simulink model "URM_IGM_2b"  (R2014a)
settings: Solver=ode45  StartTime=0.0  StopTime=inf  RelTol=1e-3
values from neighbouring files (symbols this model uses):
  a1 = 2    [URM_SP.m]
  a2 = 1.5    [URM_SP.m]
  a3 = 0.5    [URM_SP.m]
  D = linspace(d1,d2,n)    [URM_SP.m]
libraries: mblibv1 x12, simulink x3
settings Model: Creator=kajak_000  LastModifiedBy=kajak_000
settings SimMechanicsCC: VisDuringSimulation=on

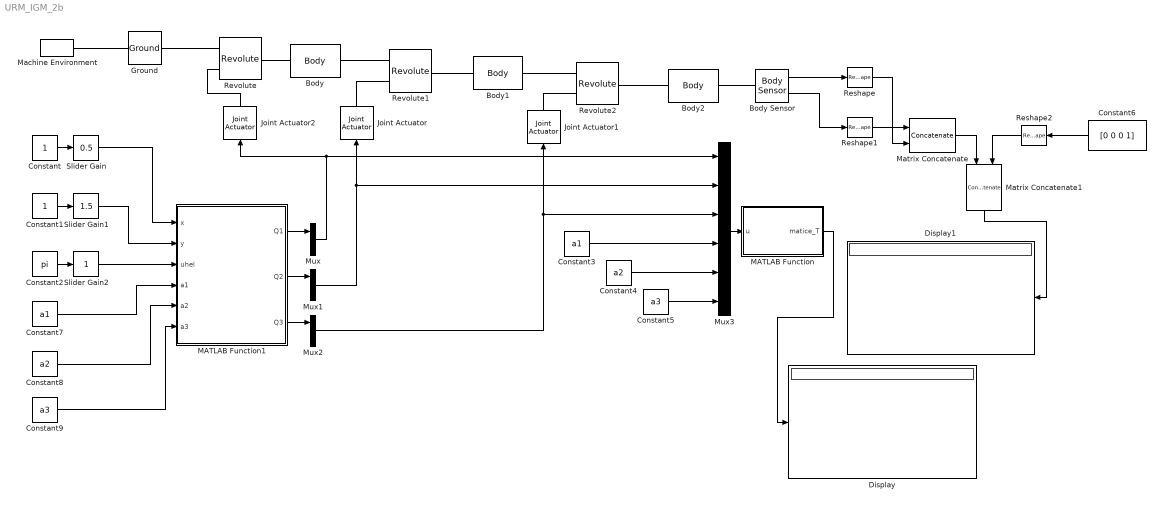
== system URM_IGM_2b ==
  Body : mblibv1/Bodies/Body  LConnTagsString=CS1  RConnTagsString=CS2  UpdateFromCAD=off  DialogClass=MechanicalBodyBlock  Mass=1  MassUnits=kg  InertiaUnits=kg*m^2  Inertia=eye(3)  Shape=Cylinder  ShapeDims=[1 1]  ShapeUnits=m  ShapeUse=false  Density=1  DensityUnits=kg/m^3  DensityUse=false  GraphicsMode=MACHINE_DEFAULT  BodyColorSelMode=MACHINE_DEFAULT  BodyColor=[1 0 0]  AttachedToCS=CG  CG=Left$CG$rameno1.CG$WORLD$WORLD$m$[0 0 0]$Euler X-Y-Z$deg$WORLD$false$none  WorkingFrames=Left$CS1$rameno1.A$World$World$m$[0 0 0]$Euler X-Y-Z$deg$WORLD$true$none#Right$CS2$rameno1.B$World$World$m$[0 0 0]$Euler X-Y-Z$deg$WORLD$true$none  CGPos=rameno1.CG  CGRot=[0 0 0]  CS0Pos=[]  CS0Rot=[]  CS1Pos=rameno1.A  CS1Rot=[0 0 0]  CS2Pos=rameno1.B  CS2Rot=[0 0 0]  CS3Pos=[]  CS3Rot=[]  CS4Pos=[]  CS4Rot=[]  CS5Pos=[]  CS5Rot=[]  CS6Pos=[]  CS6Rot=[]  CS7Pos=[]  CS7Rot=[]  CS8Pos=[]  CS8Rot=[]  CS9Pos=[]  CS9Rot=[]  CS10Pos=[]  CS10Rot=[]  CS11Pos=[]  CS11Rot=[]  CS12Pos=[]  CS12Rot=[]  CS13Pos=[]  CS13Rot=[]  CS14Pos=[]  CS14Rot=[]  CS15Pos=[]  CS15Rot=[]  CS16Pos=[]  CS16Rot=[]  CS17Pos=[]  CS17Rot=[]  CS18Pos=[]  CS18Rot=[]  CS19Pos=[]  CS19Rot=[]  CS20Pos=[]  CS20Rot=[]
  Body Sensor : mblibv1/Sensors &  Actuators/Body Sensor  UpdateFromCAD=off  PhysicalDomain=Mechanical  PortType=blob  Muxed=off  Pose=on  Angle=on  AngleUnits=deg  ArcVelocity=off  ArcVelocityUnits=deg/s  ArcAcceleration=off  ArcAccelerationUnits=deg/s^2  CoordPosition=on  CoordPositionUnits=m  Velocity=off  VelocityUnits=m/s  Acceleration=off  AccelerationUnits=m/s^2  Quaternion=on  QuaternionDT=off  QuaternionDDT=off  QuaternionUnits=off  OutputVector=[1]  ActiveIO=on  Width=12  DialogClass=MechanicalSensorBlock  ReferenceFrame=Absolute (World)
  Body1 : mblibv1/Bodies/Body  LConnTagsString=CS1  RConnTagsString=CS2  UpdateFromCAD=off  DialogClass=MechanicalBodyBlock  Mass=1  MassUnits=kg  InertiaUnits=kg*m^2  Inertia=eye(3)  Shape=Cylinder  ShapeDims=[1 1]  ShapeUnits=m  ShapeUse=false  Density=1  DensityUnits=kg/m^3  DensityUse=false  GraphicsMode=MACHINE_DEFAULT  BodyColorSelMode=MACHINE_DEFAULT  BodyColor=[1 0 0]  AttachedToCS=CG  CG=Left$CG$rameno2.CG$WORLD$WORLD$m$[0 0 0]$Euler X-Y-Z$deg$WORLD$false$none  WorkingFrames=Left$CS1$rameno2.A$World$World$m$[0 0 0]$Euler X-Y-Z$deg$WORLD$true$none#Right$CS2$rameno2.B$World$World$m$[0 0 0]$Euler X-Y-Z$deg$WORLD$true$none  CGPos=rameno2.CG  CGRot=[0 0 0]  CS0Pos=[]  CS0Rot=[]  CS1Pos=rameno2.A  CS1Rot=[0 0 0]  CS2Pos=rameno2.B  CS2Rot=[0 0 0]  CS3Pos=[]  CS3Rot=[]  CS4Pos=[]  CS4Rot=[]  CS5Pos=[]  CS5Rot=[]  CS6Pos=[]  CS6Rot=[]  CS7Pos=[]  CS7Rot=[]  CS8Pos=[]  CS8Rot=[]  CS9Pos=[]  CS9Rot=[]  CS10Pos=[]  CS10Rot=[]  CS11Pos=[]  CS11Rot=[]  CS12Pos=[]  CS12Rot=[]  CS13Pos=[]  CS13Rot=[]  CS14Pos=[]  CS14Rot=[]  CS15Pos=[]  CS15Rot=[]  CS16Pos=[]  CS16Rot=[]  CS17Pos=[]  CS17Rot=[]  CS18Pos=[]  CS18Rot=[]  CS19Pos=[]  CS19Rot=[]  CS20Pos=[]  CS20Rot=[]
  Body2 : mblibv1/Bodies/Body  LConnTagsString=CS1  RConnTagsString=CS2  UpdateFromCAD=off  DialogClass=MechanicalBodyBlock  Mass=1  MassUnits=kg  InertiaUnits=kg*m^2  Inertia=eye(3)  Shape=Cylinder  ShapeDims=[1 1]  ShapeUnits=m  ShapeUse=false  Density=1  DensityUnits=kg/m^3  DensityUse=false  GraphicsMode=MACHINE_DEFAULT  BodyColorSelMode=MACHINE_DEFAULT  BodyColor=[1 0 0]  AttachedToCS=CG  CG=Left$CG$rameno3.CG$WORLD$WORLD$m$[0 0 0]$Euler X-Y-Z$deg$WORLD$false$none  WorkingFrames=Left$CS1$rameno3.A$World$World$m$[0 0 0]$Euler X-Y-Z$deg$WORLD$true$none#Right$CS2$rameno3.B$World$World$m$[0 0 0]$Euler X-Y-Z$deg$WORLD$true$none  CGPos=rameno3.CG  CGRot=[0 0 0]  CS0Pos=[]  CS0Rot=[]  CS1Pos=rameno3.A  CS1Rot=[0 0 0]  CS2Pos=rameno3.B  CS2Rot=[0 0 0]  CS3Pos=[]  CS3Rot=[]  CS4Pos=[]  CS4Rot=[]  CS5Pos=[]  CS5Rot=[]  CS6Pos=[]  CS6Rot=[]  CS7Pos=[]  CS7Rot=[]  CS8Pos=[]  CS8Rot=[]  CS9Pos=[]  CS9Rot=[]  CS10Pos=[]  CS10Rot=[]  CS11Pos=[]  CS11Rot=[]  CS12Pos=[]  CS12Rot=[]  CS13Pos=[]  CS13Rot=[]  CS14Pos=[]  CS14Rot=[]  CS15Pos=[]  CS15Rot=[]  CS16Pos=[]  CS16Rot=[]  CS17Pos=[]  CS17Rot=[]  CS18Pos=[]  CS18Rot=[]  CS19Pos=[]  CS19Rot=[]  CS20Pos=[]  CS20Rot=[]
  Constant : Constant
  Constant1 : Constant
  Constant2 : Constant  Value=pi
  Constant3 : Constant  Value=a1
  Constant4 : Constant  Value=a2
  Constant5 : Constant  Value=a3
  Constant6 : Constant  Value=[0 0 0 1]
  Constant7 : Constant  Value=a1
  Constant8 : Constant  Value=a2
  Constant9 : Constant  Value=a3
  Display : Display
  Display1 : Display
  Ground : mblibv1/Bodies/Ground  UpdateFromCAD=off  LeftPortType=env  RightPortType=workingframe  PhysicalDomain=Mechanical  DialogClass=GroundBlock  CoordPosition=rameno1.A  CoordPositionUnits=m  StateVectorMgrId=2  MachineId=[3 0]  ShowEnvPort=on  ParameterChecksum=[1855432710, 246202875, 3894951907, 3251133505]  TopologyChecksum=[2388364943, 139228797, 3181585862, 3949180252]
  Joint Actuator : mblibv1/Sensors &  Actuators/Joint Actuator  UpdateFromCAD=off  PhysicalDomain=Mechanical  PortType=blob  ActuationStyle=Motion  AngleUnits=rad  ArcVelocityUnits=rad/s  ArcAccelerationUnits=rad/s^2  CoordPositionUnits=m  VelocityUnits=m/s  AccelerationUnits=m/s^2  ForceUnits=N  TorqueUnits=N*m  ActiveIO=on  Width=3  DialogClass=MechanicalActuatorBlock  Primitive=R1  ReferenceFrame=Absolute (World)
  Joint Actuator1 : mblibv1/Sensors &  Actuators/Joint Actuator  UpdateFromCAD=off  PhysicalDomain=Mechanical  PortType=blob  ActuationStyle=Motion  AngleUnits=rad  ArcVelocityUnits=rad/s  ArcAccelerationUnits=rad/s^2  CoordPositionUnits=m  VelocityUnits=m/s  AccelerationUnits=m/s^2  ForceUnits=N  TorqueUnits=N*m  ActiveIO=on  Width=3  DialogClass=MechanicalActuatorBlock  Primitive=R1  ReferenceFrame=Absolute (World)
  Joint Actuator2 : mblibv1/Sensors &  Actuators/Joint Actuator  UpdateFromCAD=off  PhysicalDomain=Mechanical  PortType=blob  ActuationStyle=Motion  AngleUnits=rad  ArcVelocityUnits=rad/s  ArcAccelerationUnits=rad/s^2  CoordPositionUnits=m  VelocityUnits=m/s  AccelerationUnits=m/s^2  ForceUnits=N  TorqueUnits=N*m  ActiveIO=on  Width=3  DialogClass=MechanicalActuatorBlock  Primitive=R1  ReferenceFrame=Absolute (World)
  MATLAB Function : MATLAB Function  TreatAsAtomicUnit=on
  MATLAB Function1 : MATLAB Function  TreatAsAtomicUnit=on
  Machine Environment : mblibv1/Bodies/Machine Environment  PortType=env  PhysicalDomain=Mechanical  DialogTemplateClass=MECH.MachineEnvironment  SyncWhenCopied=off  Gravity=[0 0 0]  GravityUnits=m/s^2  GravityAsSignal=off  Dimensionality=Auto-detect  AnalysisType=Forward dynamics  LinearAssemblyTolerance=1e-3  LinearAssemblyToleranceUnits=m  AngularAssemblyTolerance=1e-3  AngularAssemblyToleranceUnits=rad  ConstraintSolverType=Stabilizing  ConstraintRelTolerance=1e-4  ConstraintAbsTolerance=1e-4  UseRobustSingularityHandling=off  RedundancyAnalysisToleranceType=Automatically select tolerance  RedundancyAnalysisTolerance=1e-14  StatePerturbationType=Fixed  PerturbationSize=1e-5  VisualizeMachine=on  BodyVisualizationType=Use model default body geometries  BodyColorSelMode=Use model default  DefaultBodyColor=[1 0 0]
  Matrix Concatenate : Concatenate  Mode=Multidimensional array  ConcatenateDimension=2
  Matrix Concatenate1 : Concatenate  Mode=Multidimensional array
  Mux : Mux  Inputs=3
  Mux1 : Mux  Inputs=3
  Mux2 : Mux  Inputs=3
  Mux3 : Mux  Inputs=6
  Reshape : Reshape  OutputDimensionality=Column vector (2-D)
  Reshape1 : Reshape  OutputDimensionality=Customize  OutputDimensions=[3,3]
  Reshape2 : Reshape  OutputDimensionality=Row vector (2-D)  OutputDimensions=[3,1]
  Revolute : mblibv1/Joints/Revolute  LConnTagsString=__newl0|SA1  RConnTagsString=__newr0  UpdateFromCAD=off  NumSAPorts=1  CutJoint=off  MarkAsCut=off  Primitives=prismatic  PrimitiveProps=R1$World$rameno1.osa$revolute  DialogClass=JointBlock  R1Axis=rameno1.osa
  Revolute1 : mblibv1/Joints/Revolute  LConnTagsString=__newl0|SA1  RConnTagsString=__newr0  UpdateFromCAD=off  NumSAPorts=1  CutJoint=off  MarkAsCut=off  Primitives=prismatic  PrimitiveProps=R1$World$rameno2.osa$revolute  DialogClass=JointBlock  R1Axis=rameno2.osa
  Revolute2 : mblibv1/Joints/Revolute  LConnTagsString=__newl0|SA1  RConnTagsString=__newr0  UpdateFromCAD=off  NumSAPorts=1  CutJoint=off  MarkAsCut=off  Primitives=prismatic  PrimitiveProps=R1$World$rameno3.osa$revolute  DialogClass=JointBlock  R1Axis=rameno3.osa
  Slider Gain : simulink/Math Operations/Slider Gain  low=-3  gain=0.5  high=3
  Slider Gain1 : simulink/Math Operations/Slider Gain  low=-3  gain=1.5  high=3
  Slider Gain2 : simulink/Math Operations/Slider Gain  low=-5  gain=1  high=5
  wires:
  Slider Gain/1 -> MATLAB Function1/1(x)
  Constant/1 -> Slider Gain/1
  Constant1/1 -> Slider Gain1/1
  Constant2/1 -> Slider Gain2/1
  Constant3/1 -> Mux3/4
  Constant4/1 -> Mux3/5
  Constant5/1 -> Mux3/6
  Mux3/1 -> MATLAB Function/1(u)
  MATLAB Function/1(matice_T) -> Display/1
  Body Sensor/1 -> Reshape/1
  Body Sensor/2 -> Reshape1/1
  Reshape1/1 -> Matrix Concatenate/1
  Reshape/1 -> Matrix Concatenate/2
  Constant6/1 -> Reshape2/1
  Matrix Concatenate/1 -> Matrix Concatenate1/1
  Reshape2/1 -> Matrix Concatenate1/2
  Matrix Concatenate1/1 -> Display1/1
  Slider Gain1/1 -> MATLAB Function1/2(y)
  Slider Gain2/1 -> MATLAB Function1/3(uhel)
  Constant7/1 -> MATLAB Function1/4(a1)
  Constant8/1 -> MATLAB Function1/5(a2)
  Constant9/1 -> MATLAB Function1/6(a3)
  MATLAB Function1/1(Q1) -> Mux/1
  MATLAB Function1/2(Q2) -> Mux1/1
  MATLAB Function1/3(Q3) -> Mux2/1
  Mux/1 -> Joint Actuator2/1, Mux3/1
  Mux1/1 -> Joint Actuator/1, Mux3/2
  Mux2/1 -> Mux3/3, Joint Actuator1/1
  connections:
  Machine Environment/RConn1 -- Ground/LConn1
  Ground/RConn1 -- Revolute/LConn1
  Revolute/RConn1 -- Body/LConn1
  Body/RConn1 -- Revolute1/LConn1
  Revolute1/RConn1 -- Body1/LConn1
  Body1/RConn1 -- Revolute2/LConn1
  Revolute2/RConn1 -- Body2/LConn1
  Body2/RConn1 -- Body Sensor/LConn1
  Joint Actuator/RConn1 -- Revolute1/LConn2
  Joint Actuator1/RConn1 -- Revolute2/LConn2
  Joint Actuator2/RConn1 -- Revolute/LConn2

== matlab function URM_IGM_2b/MATLAB Function1 ==
  data: x input; y input; uhel input; a1 input; a2 input; a3 input; Q1 output; Q2 output; Q3 output
function [Q1, Q2, Q3] = IGM_funkce( x, y, uhel, a1, a2, a3)
% Q2
    cosQ2 = ((x - a3 * cos(uhel))^2 + (y - a3 * sin(uhel))^2 - a2^2 - a1^2)/(2*a1*a2);
    sinQ2 = - abs( sqrt(1 - cosQ2)); %reseni +-
    
    Q2 = atan2(sinQ2, cosQ2);
% Q1
    A = [-a2 * sinQ2, a2*cosQ2 + a1;
         a2 * cosQ2 + a1, -a2*sinQ2];
    B = [x - a3 * cos(uhel); y - a3 * sin(uhel)];
    V = A^(-1) * B;
    sinQ1 = V(1);
    cosQ1 = V(2);
    
    Q1 = atan2(sinQ1, cosQ1);
% Q3
    
    Q3 = uhel - Q2 - Q1;
end

== matlab function URM_IGM_2b/MATLAB Function ==
  data: u input; matice_T output
function matice_T = DGM_funkce(u)
Q1 = u(1);
Q2 = u(4);
Q3 = u(7);
a1 = u(10);
a2 = u(11);
a3 = u(12);
matice_T = zeros(4);

x = a3 * cos(Q1 + Q2 + Q3) + a2 * cos(Q1 + Q2) + a1 * cos(Q1);
y = a3 * sin(Q1 + Q2 + Q3) + a2 * sin(Q1 + Q2) + a1 * sin(Q1);
vysledny_uhel = Q1 + Q2 + Q3; 

matice_T = [ cos(vysledny_uhel),-sin(vysledny_uhel),0,x;
            sin(vysledny_uhel),cos(vysledny_uhel),0,y;
            0,0,1,0;
            0,0,0,1 ];
end
